simulink model "augmented_closedloop"  (R2019b)
settings: Solver=VariableStepAuto  StartTime=0.0  StopTime=10.0  RelTol=1e-3
values from neighbouring files (symbols this model uses):
  A = A*(v_phi(k,i)*s^i)    [Roberts_Q_design.m]    (also in main_fmincon.m = []; rocket_model.m = [0,1,0,0,0,0; ss_model.mat = [0  0; 1  0]; verif.m = [0,1;0,0])
  B = B*(s-alpha(i))    [Roberts_Q_design.m]    (also in controller_design.m = B*C(2); main_yp_fminunc.m = B*C(2); rocket_controllerdesign.m = B*C(2); rocket_controllerdesign_z.m = B*C(2))
  C = [0,1]    [controller_design.m]    (also in main_yp_fminunc.m; rocket_controllerdesign.m; rocket_controllerdesign_z.m; rocket_model.m = eye(6))
  D = 0    [rocket_model.m]    (also in ss_model.mat; verif.m)
  K = minreal(Q/(1+Q*P))    [cost.m]    (also in cost_LQ.m = tf((conv(denQ{1},numK0{1})+conv(numQ{1},den_sys{1})),(conv(d; cost_con.m = tf((conv(denQ{1},numK0{1})+conv(numQ{1},den_sys{1})),(conv(d; cost_disturb.m = tf((conv(denQ{1},numK0{1})+conv(numQ{1},den_sys{1})),(conv(d; fminunc_LQ.m = tf((conv(denQ{1},numK0{1})+conv(numQ{1},den_sys{1})),(conv(d)
  L = lqe(A,G,C,Qe,Re)    [controller_design.m]    (also in main_yp_fminunc.m; rocket_controllerdesign.m; rocket_controllerdesign_z.m; rocket_model.m)
undefined symbols (not defined in the file or in its folder): AQ, BQ, CQ, DQ
settings Model: Creator=bia  LastModifiedBy=bia

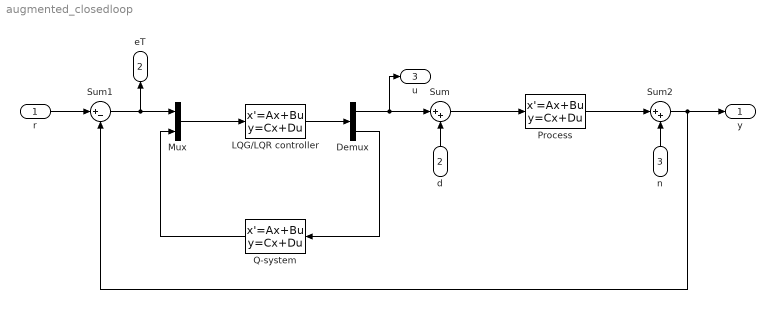
== system augmented_closedloop ==
  r : Inport
  d : Inport  Port=2
  n : Inport  Port=3
  Demux : Demux  Outputs=2
  LQG/LQR controller : StateSpace  A=A-L*C-B*K  B=[-L,B]  C=-K  D=[1,1]  InitialCondition=0
  Mux : Mux  Inputs=2
  "Process " : StateSpace  A=A  B=B  C=C  D=D  InitialCondition=0
  Q-system : StateSpace  A=AQ  B=BQ  C=CQ  D=DQ  InitialCondition=0
  Sum : Sum  Inputs=|++
  Sum1 : Sum  Inputs=|+-
  Sum2 : Sum  Inputs=|++
  y : Outport
  eT : Outport  Port=2
  u : Outport  Port=3
  wires:
  Mux/1 -> LQG/LQR controller/1
  LQG/LQR controller/1 -> Demux/1
  Sum1/1 -> eT/1, Mux/1
  Demux/2 -> Q-system/1
  Demux/1 -> u/1, Sum/1
  Sum/1 -> "Process "/1
  "Process "/1 -> Sum2/1
  Q-system/1 -> Mux/2
  r/1 -> Sum1/1
  d/1 -> Sum/2
  n/1 -> Sum2/2
  Sum2/1 -> Sum1/2, y/1
